simulink model "AUV_Model"  (R2020a)
settings: Solver=VariableStepAuto  StartTime=0.0  StopTime=T  FixedStep=0.5  RelTol=1e-3
InitFcn:
  | mdlWks = get_param(gcs,'ModelWorkspace');
  | a = getVariable(mdlWks,'a');
  | b = getVariable(mdlWks,'b');
  | c = getVariable(mdlWks,'c');
StopFcn:
  | %figure(2)
  | %plot3(Position_Data(1,1),Position_Data(1,2),Position_Data(1,3),'r*')
  | %hold on
  | %plot3(Position_Data(:,1),Position_Data(:,2),Position_Data(:,3));
  | %plot3(Position_Data(end,1),Position_Data(end,2),Position_Data(end,3),'g*');
  | %grid on
  | %legend('Start Point','Trajectory','End Point')
model workspace (MAT data in the model file):
  a = 0
  b = 1
  c = 1
values from neighbouring files (symbols this model uses):
  Ts = 0.1    [plant_init.m]
libraries: dspfdesign x6, mpclib x1, aerolibnav x1
(part 2 of 2)

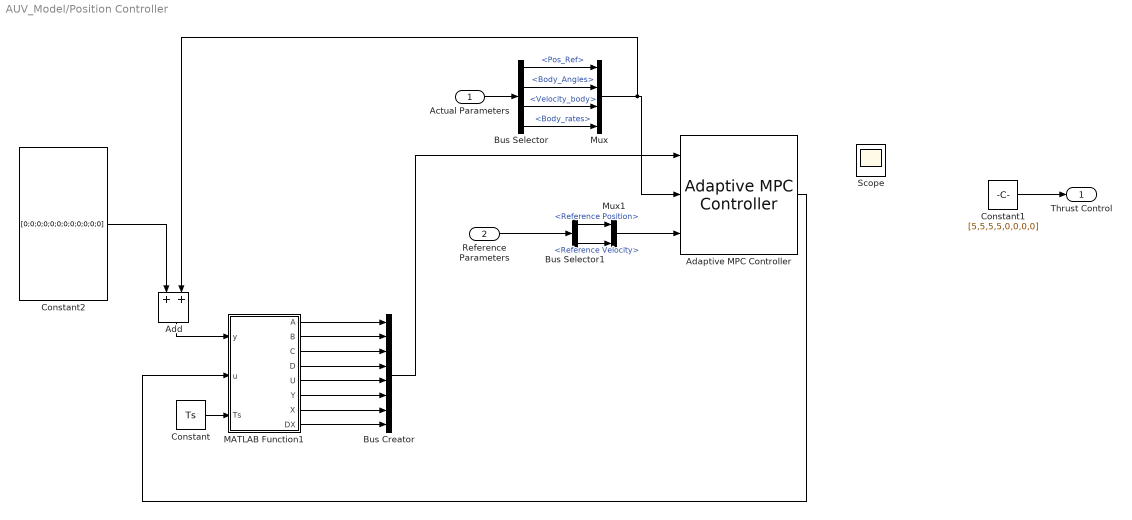
== system AUV_Model/Position Controller ==
  Actual Parameters : Inport
  Reference Parameters : Inport  Port=2
  Adaptive MPC Controller : mpclib/Adaptive MPC Controller  SCDEnableBlockLinearizationSpecification=on  mpcobj=mpcobj  x0=x  enable_value=0  updateMPCinCallerWorkspace=on  md_inport=off  mv_inport=off  uref_inport=off  return_cost=off  return_mvseq=off  return_qpstatus=off  return_xseq=off  return_state=off  return_ovseq=off  state_inport=off  isltv_plant=off  umin_inport=off  umax_inport=off  ymin_inport=off  ymax_inport=off  cc_inport=off  ywt_inport=off  uwt_inport=off  duwt_inport=off  rhoeps_inport=off  pm_inport=off  MaximumP=10  HorizonChoice=FixedHorizon  BlockDataType=double  SampleTimeInherited=off  switch_inport=off
  Add : Sum
  Bus Creator : BusCreator  Inputs=8
  Bus Selector : BusSelector  OutputSignals=Pos_Ref,Body_Angles,Velocity_body,Body_rates
  Bus Selector1 : BusSelector  OutputSignals=Reference Position,Reference Velocity
  Constant : Constant  Value=Ts
  Constant1 : Constant  Value=[5,5,5,5,0,0,0,0]
  Constant2 : Constant  Value=[0;0;0;0;0;0;0;0;0;0;0;0]  VectorParams1D=off
  MATLAB Function1 : MATLAB Function  TreatAsAtomicUnit=on
  Mux : Mux
  Mux1 : Mux  Inputs=2
  Scope : Scope
  Thrust Control : Outport  VectorParamsAs1DForOutWhenUnconnected=off
  wires:
  Actual Parameters/1 -> Bus Selector/1
  Bus Selector/1 -> Mux/1  "<Pos_Ref>"
  Bus Selector/2 -> Mux/2  "<Body_Angles>"
  Bus Selector1/1 -> Mux1/1  "<Reference Position>"
  Reference Parameters/1 -> Bus Selector1/1
  Bus Selector1/2 -> Mux1/2  "<Reference Velocity>"
  Bus Selector/3 -> Mux/3  "<Velocity_body>"
  Bus Selector/4 -> Mux/4  "<Body_rates>"
  Mux1/1 -> Adaptive MPC Controller/3
  Mux/1 -> Add/2, Adaptive MPC Controller/2
  MATLAB Function1/8(DX) -> Bus Creator/8
  MATLAB Function1/5(U) -> Bus Creator/5
  Add/1 -> MATLAB Function1/1(y)
  MATLAB Function1/6(Y) -> Bus Creator/6
  MATLAB Function1/7(X) -> Bus Creator/7
  Constant2/1 -> Add/1
  Adaptive MPC Controller/1 -> MATLAB Function1/2(u)
  MATLAB Function1/4(D) -> Bus Creator/4
  MATLAB Function1/2(B) -> Bus Creator/2
  MATLAB Function1/3(C) -> Bus Creator/3
  MATLAB Function1/1(A) -> Bus Creator/1
  Constant/1 -> MATLAB Function1/3(Ts)
  Bus Creator/1 -> Adaptive MPC Controller/1
  Constant1/1 -> Thrust Control/1

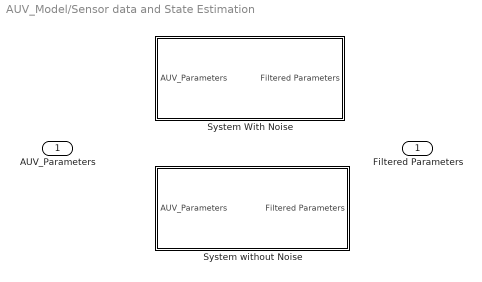
== system AUV_Model/Sensor data and State Estimation ==
  AUV_Parameters : Inport
  System With Noise : Subsystem  VariantControl=b==0
  System without Noise : Subsystem  VariantControl=b==1
  Filtered Parameters : Outport  VectorParamsAs1DForOutWhenUnconnected=off

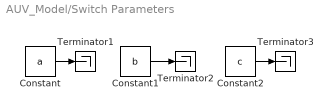
== system AUV_Model/Switch Parameters ==
  Constant : Constant  Value=a
  Constant1 : Constant  Value=b
  Constant2 : Constant  Value=c
  Terminator1 : Terminator
  Terminator2 : Terminator
  Terminator3 : Terminator
  wires:
  Constant/1 -> Terminator1/1
  Constant1/1 -> Terminator2/1
  Constant2/1 -> Terminator3/1

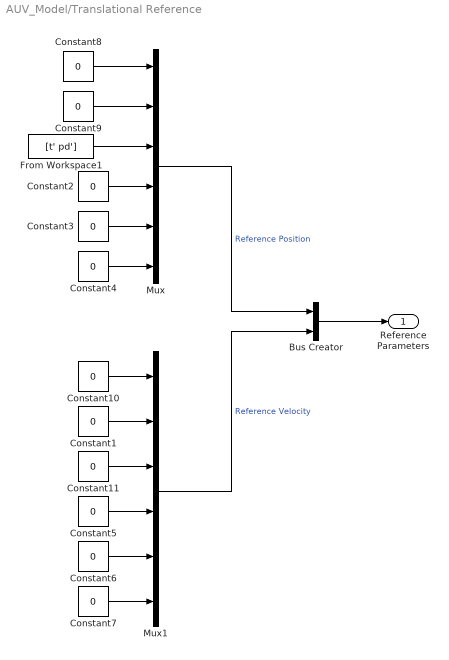
== system AUV_Model/Translational Reference ==
  Bus Creator : BusCreator  Inputs=2
  Constant{1..11} (11 alike) : Constant  Value=0
  From Workspace1 : FromWorkspace  VariableName=[t' pd']
  Mux : Mux  Inputs=6
  Mux1 : Mux  Inputs=6
  Reference Parameters : Outport  VectorParamsAs1DForOutWhenUnconnected=off
  wires:
  Mux/1 -> Bus Creator/1  "Reference Position"
  Mux1/1 -> Bus Creator/2  "Reference Velocity"
  Bus Creator/1 -> Reference Parameters/1
  Constant1/1 -> Mux1/2
  Constant2/1 -> Mux/4
  Constant3/1 -> Mux/5
  Constant4/1 -> Mux/6
  Constant6/1 -> Mux1/5
  Constant7/1 -> Mux1/6
  Constant5/1 -> Mux1/4
  Constant9/1 -> Mux/2
  Constant10/1 -> Mux1/1
  Constant11/1 -> Mux1/3
  From Workspace1/1 -> Mux/3
  Constant8/1 -> Mux/1

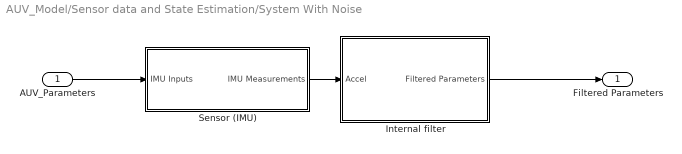
== system AUV_Model/Sensor data and State Estimation/System With Noise ==
  AUV_Parameters : Inport
  " Sensor (IMU)" : Subsystem
  Internal filter : Subsystem
  Filtered Parameters : Outport  VectorParamsAs1DForOutWhenUnconnected=off
  wires:
  AUV_Parameters/1 -> " Sensor (IMU)"/1(IMU Inputs)
  Internal filter/1(Filtered Parameters) -> Filtered Parameters/1
  " Sensor (IMU)"/1(IMU Measurements) -> Internal filter/1(Accel)

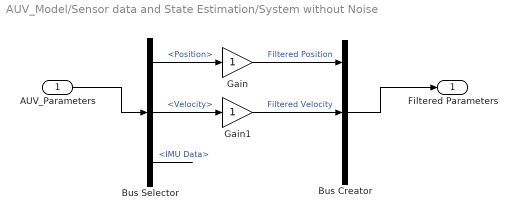
== system AUV_Model/Sensor data and State Estimation/System without Noise ==
  AUV_Parameters : Inport
  Bus Creator : BusCreator  Inputs=3
  Bus Selector : BusSelector  OutputSignals=Position,Velocity,IMU Data
  Gain : Gain
  Gain1 : Gain
  Filtered Parameters : Outport  VectorParamsAs1DForOutWhenUnconnected=off
  wires:
  Bus Creator/1 -> Filtered Parameters/1
  Bus Selector/2 -> Gain1/1  "<Velocity>"
  Bus Selector/1 -> Gain/1  "<Position>"
  Gain1/1 -> Bus Creator/2  "Filtered Velocity"
  Gain/1 -> Bus Creator/1  "Filtered Position"
  AUV_Parameters/1 -> Bus Selector/1
  Bus Selector/3 -> ?  "<IMU Data>"

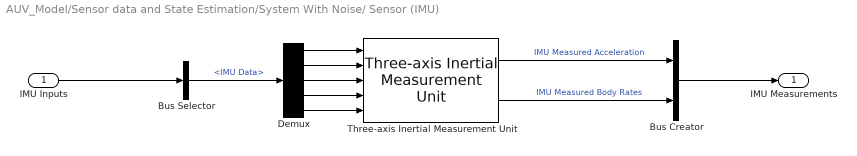
== system AUV_Model/Sensor data and State Estimation/System With Noise/ Sensor (IMU) ==
  IMU Inputs : Inport
  Bus Creator : BusCreator  Inputs=2
  Bus Selector : BusSelector  OutputSignals=IMU Data
  Demux : Demux  Outputs=5
  Three-axis Inertial Measurement Unit : aerolibnav/Three-axis Inertial Measurement Unit  units=Metric (MKS)  imu=[0 0 0]  i_Ts=0  dtype_a=on  w_a=190  z_a=0.707  a_sf_cc=[1 0 0; 0 1 0; 0 0 1]  a_bias=[0 0 0]  a_sat="[-inf  -inf  -inf  inf inf inf]"  dtype_g=on  w_g=190  z_g=0.707  g_sf_cc=[1 0 0; 0 1 0; 0 0 1]  g_bias=[0 0 0]  g_sens=[0 0 0]  g_sat="[-inf  -inf  -inf  inf inf inf]"  i_rand=on  i_seeds=[23093 23094 23095 23096 23097 23098]  i_pow=[0.00001 0.00001 0.00001 0.00001 0.00001 0.00001]
  IMU Measurements : Outport  VectorParamsAs1DForOutWhenUnconnected=off
  wires:
  Three-axis Inertial Measurement Unit/1 -> Bus Creator/1  "IMU Measured Acceleration"
  Demux/2 -> Three-axis Inertial Measurement Unit/2
  Demux/4 -> Three-axis Inertial Measurement Unit/4
  Demux/5 -> Three-axis Inertial Measurement Unit/5
  Demux/3 -> Three-axis Inertial Measurement Unit/3
  Demux/1 -> Three-axis Inertial Measurement Unit/1
  Three-axis Inertial Measurement Unit/2 -> Bus Creator/2  "IMU Measured Body Rates"
  IMU Inputs/1 -> Bus Selector/1
  Bus Selector/1 -> Demux/1  "<IMU Data>"
  Bus Creator/1 -> IMU Measurements/1

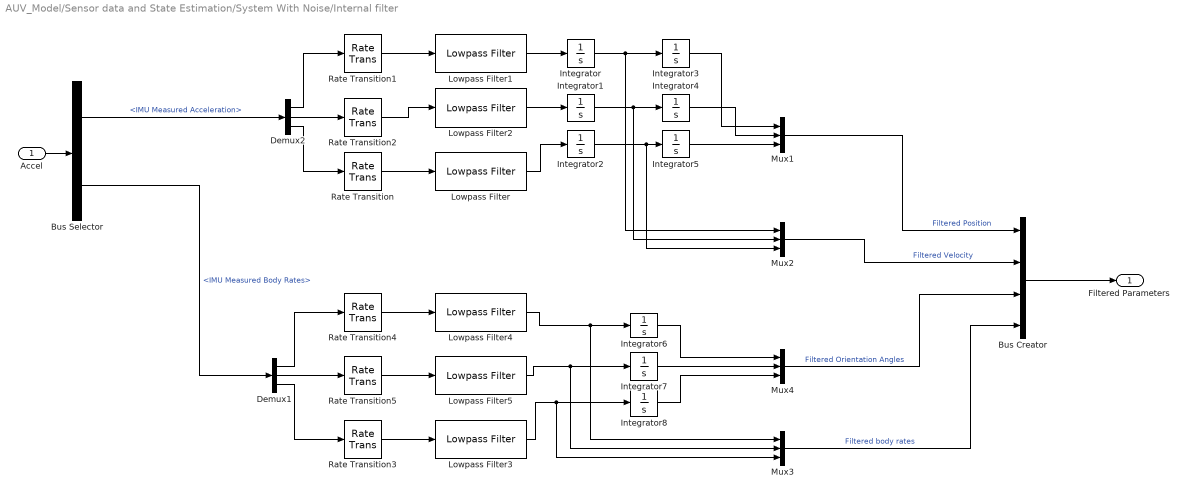
== system AUV_Model/Sensor data and State Estimation/System With Noise/Internal filter ==
  Accel : Inport
  Bus Creator : BusCreator  Inputs=4
  Bus Selector : BusSelector  OutputSignals=IMU Measured Acceleration,IMU Measured Body Rates
  Demux1 : Demux  Outputs=3
  Demux2 : Demux  Outputs=3
  Integrator{,1..8} (9 alike) : Integrator
  Lowpass Filter{,1..5} (6 alike) : dspfdesign/Lowpass Filter  FilterType=FIR  DesignForMinimumOrder=on  FilterOrder=50  PassbandFrequency=1/100  StopbandFrequency=45  PassbandRipple=0.1  StopbandAttenuation=80  InheritSampleRate=off  SampleRate=100  SimulateUsing=Interpreted execution  roundingMode=Floor  coeffsDataTypeStr=fixdt(1,16)
  Mux{1..4} (4 alike) : Mux  Inputs=3
  Rate Transition{,1..5} (6 alike) : RateTransition  OutPortSampleTime=0.01
  Filtered Parameters : Outport  VectorParamsAs1DForOutWhenUnconnected=off
  wires:
  Rate Transition5/1 -> Lowpass Filter5/1
  Rate Transition4/1 -> Lowpass Filter4/1
  Demux1/1 -> Rate Transition4/1
  Lowpass Filter3/1 -> Mux3/3, Integrator8/1
  Demux1/2 -> Rate Transition5/1
  Lowpass Filter5/1 -> Mux3/2, Integrator7/1
  Lowpass Filter4/1 -> Mux3/1, Integrator6/1
  Integrator6/1 -> Mux4/1
  Rate Transition3/1 -> Lowpass Filter3/1
  Integrator8/1 -> Mux4/3
  Demux1/3 -> Rate Transition3/1
  Integrator7/1 -> Mux4/2
  Accel/1 -> Bus Selector/1
  Bus Selector/1 -> Demux2/1  "<IMU Measured Acceleration>"
  Bus Selector/2 -> Demux1/1  "<IMU Measured Body Rates>"
  Mux4/1 -> Bus Creator/3  "Filtered Orientation Angles"
  Mux3/1 -> Bus Creator/4  "Filtered body rates"
  Bus Creator/1 -> Filtered Parameters/1
  Integrator2/1 -> Integrator5/1, Mux2/3
  Integrator/1 -> Mux2/1, Integrator3/1
  Mux2/1 -> Bus Creator/2  "Filtered Velocity"
  Mux1/1 -> Bus Creator/1  "Filtered Position"
  Lowpass Filter/1 -> Integrator2/1
  Demux2/2 -> Rate Transition2/1
  Rate Transition1/1 -> Lowpass Filter1/1
  Integrator4/1 -> Mux1/2
  Demux2/3 -> Rate Transition/1
  Lowpass Filter2/1 -> Integrator1/1
  Lowpass Filter1/1 -> Integrator/1
  Demux2/1 -> Rate Transition1/1
  Integrator5/1 -> Mux1/3
  Integrator1/1 -> Integrator4/1, Mux2/2
  Rate Transition/1 -> Lowpass Filter/1
  Integrator3/1 -> Mux1/1
  Rate Transition2/1 -> Lowpass Filter2/1

== matlab function AUV_Model/Position Controller/MATLAB Function1 ==
  data: y input; u input; A output; Ts input; B output; C output; D output; U output; Y output; X output; DX output
function [A,B,C,D,U,Y,X,DX] = Plant(y,u,Ts)
% Lineariser le model dynamique

%x=[y(4:5,1);y(7:12,1)];
%x(5)=x(5)-.85;
[Ac, Bc, Cc, Dc]=AUVStateJacobianFcn(y,u);
% Generate discrete-time model

%  nx = size(Ac,1);
%  nu = size(Bc,2);
%cplant=ss(Ac,Bc,Cc,Dc);
%plant=c2d(cplant,Ts,'zoh');

nx = size(Ac,1);
nu = size(Bc,2);
M = expm([[Ac Bc]*Ts; zeros(nu,nu+nx)]);
A = M(1:nx,1:nx);
B = M(1:nx,nx+1:nx+nu);
C = Cc;
D = Dc;
 %xx=[X(4:5,1);X(7:12)];

% cplant=ss(Ac,Bc,Cc,Dc);
% plant=c2d(cplant,Ts,'zoh');
%plant=ss(A,B,C,D,Ts);

% Nominal conditions for discrete-time plant
U=u.';
Y=(Cc*y + Dc*u).';
X=y.';
DX=(A*y+B*u-y).';
